simulink model "q_sswe"  (Simulink 7.8)
settings: Solver=ode4  StartTime=0.0  StopTime=inf  FixedStep=0.001  RelTol=1e-3  AbsTol=1e-6
values from neighbouring files (symbols this model uses):
  K = [ 0 0 0 0 0 ]    [setup_ip02_ssw.m]
  K_AMP = 1    [setup_ip02_ssw.m]
  K_EC = Pr * N_pp / ( 4 * 1024 )    (= 2.27485440932e-05)    [config_ip02.m]
  KE_SW = 2 * pi / ( 4 * 1024 )    (= 0.00153398078789)    [config_ssw.m]
  Kgs = 3    [config_ssw.m]
  MAX_I_WINDUP = 10 / 180 * pi    (= 0.174532925199)    [setup_ip02_ssw.m]
  MIN_I_WINDUP = - MAX_I_WINDUP    (= -0.174532925199)    [setup_ip02_ssw.m]
  VMAX_AMP = 2.6 * IMAX_AMP    (= 4.16)    [config_ip02.m]
  VMAX_DAC = 10    [setup_ip02_ssw.m]
  wcf = 2 * pi * 10    (= 62.8318530718)    [setup_ip02_ssw.m]
  X_LIM_ENABLE = 1    [setup_ip02_ssw.m]
  X_MAX = 0.35    [setup_ip02_ssw.m]
  X_MIN = - X_MAX    (= -0.35)    [setup_ip02_ssw.m]
  zetaf = 0.9    [setup_ip02_ssw.m]
undefined symbols (not defined in the file or in its folder): HIL, qc_get_step_size
libraries: quarc_library x7, simulink_extras x3
settings Model: Creator=MLevis  LastModifiedBy=pmartin  SimulationMode=external  ExtModeTrigDuration=10000  ExtModeAutoUpdateStatusClock=off  BufferReuse=off
settings SolverCC: PositivePriorityOrder=on
settings DataIOCC: LimitDataPoints=off
settings OptimizationCC: BooleanDataType=off  InlineInvariantSignals=on  OptimizeBlockIOStorage=off  BufferReuse=off  ExpressionFolding=off  FoldNonRolledExpr=off  LocalBlockOutputs=off  InitFltsAndDblsToZero=on
settings DebuggingCC: SaveWithParameterizedLinksMsg=none  SignalResolutionControl=TryResolveAllWithWarning  SolverPrmCheckMsg=none  MultiTaskDSMMsg=warning  MultiTaskCondExecSysMsg=none  FcnCallInpInsideContextMsg=Use local settings  StrictBusMsg=None
settings RTWCC: SystemTargetFile=quarc_windows.tlc  TemplateMakefile=quarc_default_tmf  Description=QuaRC Win32 Target  ProcessScript=quarc_windows_make_rtw_hook  IncludeERTFirstTime=on
settings STFCustomTargetCC: TargetFcnLib=ansi_tfl_tmw.mat  TargetPreCompLibLocation=C:\PROGRA~2\QUARC\lib\2011b\windows\release  SystemTargetFile=quarc_windows.tlc
settings GRTTargetCC: TargetFcnLib=ansi_tfl_tmw.mat  TargetPreCompLibLocation=C:\PROGRA~2\QUARC\lib\2011b\windows\release  ParMdlRefBuildCompliant=off  CompOptLevelCompliant=off  ConcurrentExecutionCompliant=off  MatFileLogging=off  ExtMode=on  ExtModeMexFile=quarc_comm

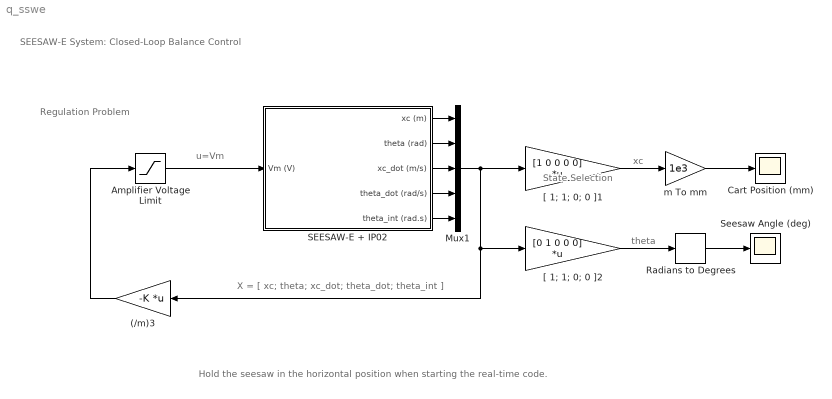
== system q_sswe ==
  note: SEESAW-E System:
      | Closed-Loop Balance Control
  note: u=Vm
  note: X = [ xc; theta; xc_dot; theta_dot; theta_int ]
  note: Regulation Problem
  note: xc
  note: State Selection
  note: theta
  note: Hold the seesaw in the horizontal position when starting the real-time code.
  (/m)3 : Gain  Gain=-K  Multiplication=Matrix(K*u)  SaturateOnIntegerOverflow=on  OutDataTypeStr=Inherit: Same as input  ParamDataTypeStr=Inherit: Same as input
  Amplifier Voltage Limit : Saturate  UpperLimit=VMAX_AMP  LowerLimit=- VMAX_AMP
  Cart Position (mm) : Scope
      settings: TickLabels=on  TimeRange=10  YMin=-250  YMax=250  SaveName=data_xc  DataFormat=Array  MaxDataPoints=10000
  Mux1 : Mux  Inputs=5
  Radians to Degrees : simulink_extras/Transformations/Radians to Degrees
  SEESAW-E + IP02 : Subsystem
  Seesaw Angle (deg) : Scope
      settings: TickLabels=on  TimeRange=10  YMin=-0.075  YMax=0.25  SaveName=data_ssw  DataFormat=Array  MaxDataPoints=10000
  "[ 1; 1; 0; 0 ]1" : Gain  Gain=[1 0 0 0 0]  Multiplication=Matrix(K*u)  SaturateOnIntegerOverflow=on  OutDataTypeStr=Inherit: Same as input  ParamDataTypeStr=Inherit: Same as input
  "[ 1; 1; 0; 0 ]2" : Gain  Gain=[0 1 0 0 0]  Multiplication=Matrix(K*u)  SaturateOnIntegerOverflow=on  OutDataTypeStr=Inherit: Same as input  ParamDataTypeStr=Inherit: Same as input
  m To mm : Gain  Gain=1e3  SaturateOnIntegerOverflow=on  OutDataTypeStr=Inherit: Same as input  ParamDataTypeStr=Inherit: Same as input
  wires:
  Amplifier Voltage Limit/1 -> SEESAW-E + IP02/1(Vm (V))
  SEESAW-E + IP02/1(xc (m)) -> Mux1/1
  SEESAW-E + IP02/4(theta_dot (rad/s)) -> Mux1/4
  Mux1/1 -> "[ 1; 1; 0; 0 ]1"/1, "[ 1; 1; 0; 0 ]2"/1, (/m)3/1
  SEESAW-E + IP02/3(xc_dot (m/s)) -> Mux1/3
  SEESAW-E + IP02/2(theta (rad)) -> Mux1/2
  m To mm/1 -> Cart Position (mm)/1
  Radians to Degrees/1 -> Seesaw Angle (deg)/1
  "[ 1; 1; 0; 0 ]2"/1 -> Radians to Degrees/1
  "[ 1; 1; 0; 0 ]1"/1 -> m To mm/1
  (/m)3/1 -> Amplifier Voltage Limit/1
  SEESAW-E + IP02/5(theta_int (rad.s)) -> Mux1/5

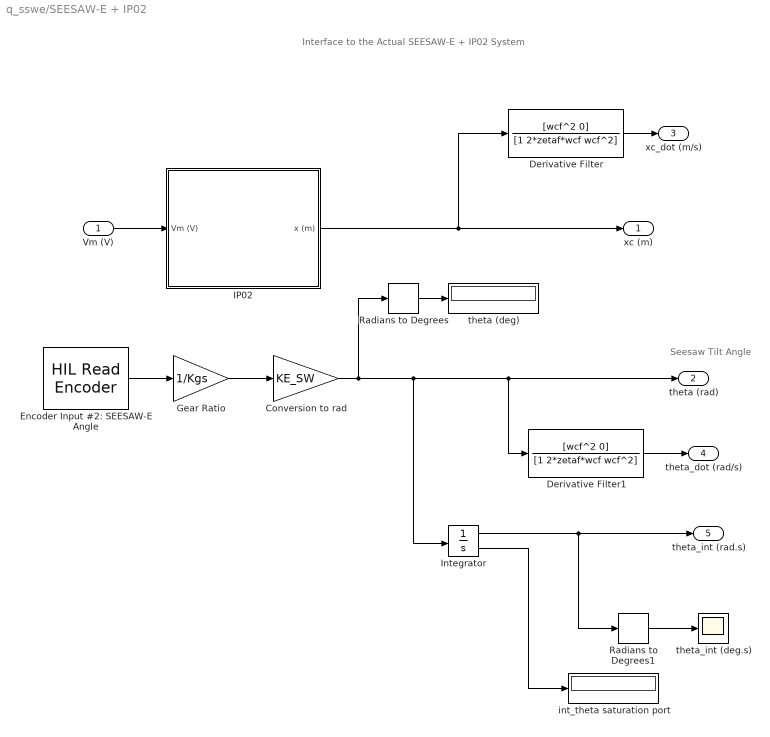
== system q_sswe/SEESAW-E + IP02 ==
  note: Interface to the Actual
      | SEESAW-E + IP02 System
  note: Seesaw Tilt Angle
  Vm (V) : Inport
  Conversion to rad : Gain  Gain=KE_SW  SaturateOnIntegerOverflow=on  OutDataTypeStr=Inherit: Same as input  ParamDataTypeStr=Inherit: Same as input
  Derivative Filter : TransferFcn  Numerator=[wcf^2 0]  Denominator=[1 2*zetaf*wcf wcf^2]
  Derivative Filter1 : TransferFcn  Numerator=[wcf^2 0]  Denominator=[1 2*zetaf*wcf wcf^2]
  Encoder Input #2: SEESAW-E Angle : quarc_library/Data Acquisition/Generic/Immediate I//O/HIL Read Encoder  object_name=HIL-1  channels=1  sample_time=qc_get_step_size  active=on  vector_output=off  data_type_mode=Inherit via back propagation  data_type=double
  Gear Ratio : Gain  Gain=1/Kgs  SaturateOnIntegerOverflow=on  OutDataTypeStr=Inherit: Same as input  ParamDataTypeStr=Inherit: Same as input
  "IP02 " : Subsystem
  Integrator : Integrator  LimitOutput=on  UpperSaturationLimit=MAX_I_WINDUP  LowerSaturationLimit=MIN_I_WINDUP  ShowSaturationPort=on
  Radians to Degrees : simulink_extras/Transformations/Radians to Degrees
  Radians to Degrees1 : simulink_extras/Transformations/Radians to Degrees
  int_theta saturation port : Display
      settings: Decimation=50
  theta (deg) : Display
      settings: Decimation=50
  theta_int (deg.s) : Scope
      settings: TickLabels=on  TimeRange=1.000000  YMin=-250  YMax=250  DataFormat=Array
  xc (m) : Outport  InitialOutput=0
  theta (rad) : Outport  Port=2  InitialOutput=0
  xc_dot (m/s) : Outport  Port=3  InitialOutput=0
  theta_dot (rad/s) : Outport  Port=4  InitialOutput=0
  theta_int (rad.s) : Outport  Port=5  InitialOutput=0
  wires:
  "IP02 "/1(x (m)) -> xc (m)/1, Derivative Filter/1
  Derivative Filter1/1 -> theta_dot (rad/s)/1
  Derivative Filter/1 -> xc_dot (m/s)/1
  Vm (V)/1 -> "IP02 "/1(Vm (V))
  Conversion to rad/1 -> Radians to Degrees/1, theta (rad)/1, Derivative Filter1/1, Integrator/1
  Radians to Degrees/1 -> theta (deg)/1
  Encoder Input #2: SEESAW-E Angle/1 -> Gear Ratio/1
  Gear Ratio/1 -> Conversion to rad/1
  Integrator/1 -> theta_int (rad.s)/1, Radians to Degrees1/1
  Integrator/2 -> int_theta saturation port/1
  Radians to Degrees1/1 -> theta_int (deg.s)/1

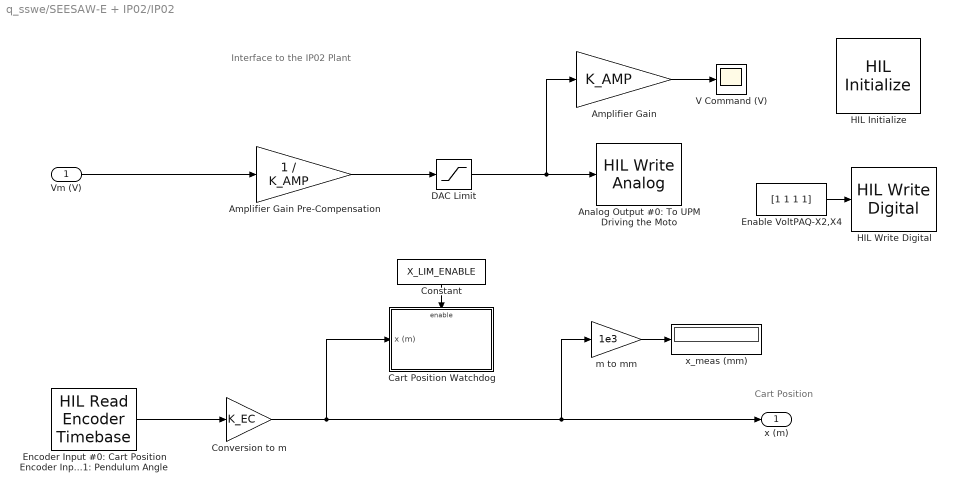
== system q_sswe/SEESAW-E + IP02/IP02  ==
  note: Cart Position
  note: Interface to the IP02 Plant
  Vm (V) : Inport
  Amplifier Gain : Gain  Gain=K_AMP  SaturateOnIntegerOverflow=on  OutDataTypeStr=Inherit: Same as input  ParamDataTypeStr=Inherit: Same as input
  Amplifier Gain Pre-Compensation : Gain  Gain=1 / K_AMP  SaturateOnIntegerOverflow=on  OutDataTypeStr=Inherit: Same as input  ParamDataTypeStr=Inherit: Same as input
  Analog Output #0: To UPM Driving the Moto : quarc_library/Data Acquisition/Generic/Immediate I//O/HIL Write Analog  Tag=unassigned  object_name=HIL-1  channels=0  sample_time=-1  active=on  vector_input=on
  Cart Position Watchdog : Subsystem  TreatAsAtomicUnit=on
  Constant : Constant  Value=X_LIM_ENABLE
  Conversion to m : Gain  Gain=K_EC  SaturateOnIntegerOverflow=on  OutDataTypeStr=Inherit: Same as input  ParamDataTypeStr=Inherit: Same as input
  DAC Limit : Saturate  UpperLimit=VMAX_DAC  LowerLimit=- VMAX_DAC
  Enable VoltPAQ-X2,X4 : Constant  Value=[1 1 1 1]
  Encoder Input #0: Cart Position Encoder Input #1: Pendulum Angle : quarc_library/Data Acquisition/Generic/Timebases/HIL Read Encoder Timebase  Tag=unassigned  object_name=HIL-1  clock=0  channels=[0]  samples_in_buffer=max(ceil(1/qc_get_step_size), 1)  active=on  vector_output=off  data_type_mode=Inherit via back propagation  data_type=double
  HIL Initialize : quarc_library/Data Acquisition/Generic/Configuration/HIL Initialize  object_name=HIL-1  board_type=q2_usb  board_number=0  board_options=d0=digital;d1=digital;led=auto;update_rate=normal  exclusive=off  active=off  hardware_clocks=[0:2]  clock_modes=[]  initial_clock_frequencies=[]  set_clock_params_at_start=off  set_clock_params_at_switch_in=off  set_clock_frequencies_at_start=off  set_clock_frequencies_at_switch_in=off  analog_input_channels=[0:1]  analog_input_maximums=10  analog_input_minimums=-10  set_analog_input_params_at_start=on  set_analog_input_params_at_switch_in=off  analog_output_channels=[0:1]  analog_output_maximums=10  analog_output_minimums=-10  initial_analog_outputs=[0]  final_analog_outputs=[0]  watchdog_analog_outputs=0  set_analog_output_params_at_start=on  set_analog_output_params_at_switch_in=off  set_analog_outputs_at_start=on  set_analog_outputs_at_switch_in=off  set_analog_outputs_at_terminate=on  set_analog_outputs_at_switch_out=off  set_analog_outputs_on_watchdog=off  digital_input_channels=[]  digital_output_channels=[0:7]  digital_output_configuration=[]  initial_digital_outputs=[0]  final_digital_outputs=[0]  watchdog_digital_outputs=[0]  set_digital_output_params_at_start=off  set_digital_output_params_at_switch_in=off  set_digital_outputs_at_start=on  set_digital_outputs_at_switch_in=off  set_digital_outputs_at_terminate=on  set_digital_outputs_at_switch_out=off  set_digital_outputs_on_watchdog=off  encoder_channels=[0:1]  quadrature=[4]  encoder_filter_frequency=[]  initial_encoder_counts=[0]  set_encoder_params_at_start=on  set_encoder_params_at_switch_in=off  set_encoder_counts_at_start=on  set_encoder_counts_at_switch_in=off  pwm_channels=[]  pwm_modes=[0]  pwm_frequency=1/0.020  pwm_configuration=[]  pwm_alignment=[]  pwm_polarity=[]  pwm_leading_deadband=[]  pwm_trailing_deadband=[]  initial_pwm_outputs=[0]  final_pwm_outputs=[0]  watchdog_pwm_outputs=[0]  set_pwm_params_at_start=on  set_pwm_params_at_switch_in=off  set_pwm_outputs_at_start=on  set_pwm_outputs_at_switch_in=off  set_pwm_outputs_at_terminate=on  set_pwm_outputs_at_switch_out=off  set_pwm_outputs_on_watchdog=off  other_output_channels=[]  initial_other_outputs=[]  final_other_outputs=[]  watchdog_other_outputs=[]  set_other_outputs_at_start=off  set_other_outputs_at_switch_in=off  set_other_outputs_at_terminate=off  set_other_outputs_at_switch_out=off  set_other_outputs_on_watchdog=off
  HIL Write Digital : quarc_library/Data Acquisition/Generic/Immediate I//O/HIL Write Digital  object_name=HIL-1  channels=[0:3]  sample_time=-1  active=off  vector_input=on
  V Command (V) : Scope
      settings: TickLabels=on  TimeRange=10  YMin=-6  YMax=6  SaveName=data_vm  DataFormat=Array  MaxDataPoints=10000
  m to mm : Gain  Gain=1e3  SaturateOnIntegerOverflow=on  OutDataTypeStr=Inherit: Same as input  ParamDataTypeStr=Inherit: Same as input
  x_meas (mm) : Display
      settings: Decimation=50
  x (m) : Outport  InitialOutput=0
  wires:
  Encoder Input #0: Cart Position Encoder Input #1: Pendulum Angle/1 -> Conversion to m/1
  Conversion to m/1 -> Cart Position Watchdog/1(x (m)), x (m)/1, m to mm/1
  Amplifier Gain Pre-Compensation/1 -> DAC Limit/1
  m to mm/1 -> x_meas (mm)/1
  Constant/1 -> Cart Position Watchdog/Enable
  DAC Limit/1 -> Analog Output #0: To UPM Driving the Moto/1, Amplifier Gain/1
  Vm (V)/1 -> Amplifier Gain Pre-Compensation/1
  Amplifier Gain/1 -> V Command (V)/1
  Enable VoltPAQ-X2,X4/1 -> HIL Write Digital/1

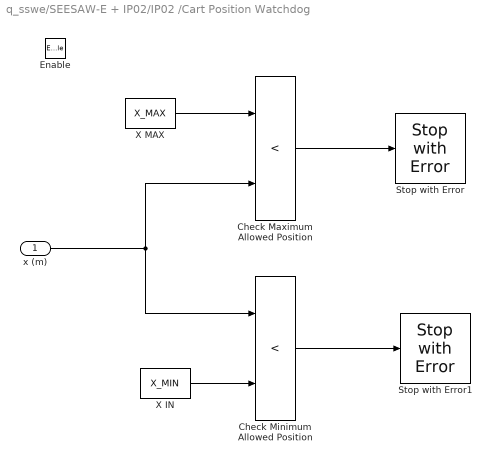
== system q_sswe/SEESAW-E + IP02/IP02 /Cart Position Watchdog ==
  x (m) : Inport
  Enable : EnablePort
  Check Maximum Allowed Position : RelationalOperator  Operator=<  InputSameDT=on
  Check Minimum Allowed Position : RelationalOperator  Operator=<  InputSameDT=on
  Stop with Error : quarc_library/Sinks/Error Handling/Stop with Error  message_type=Fixed error message  message=Maximum Limit Reached.
      settings: AttributesFormatString="\"%<message>\""
  Stop with Error1 : quarc_library/Sinks/Error Handling/Stop with Error  message_type=Fixed error message  message=Minimum Limit Reached.
      settings: AttributesFormatString="\"%<message>\""
  X IN : Constant  Value=X_MIN
  X MAX : Constant  Value=X_MAX
  wires:
  Check Maximum Allowed Position/1 -> Stop with Error/1
  x (m)/1 -> Check Minimum Allowed Position/1, Check Maximum Allowed Position/2
  X IN/1 -> Check Minimum Allowed Position/2
  Check Minimum Allowed Position/1 -> Stop with Error1/1
  X MAX/1 -> Check Maximum Allowed Position/1
